simulink model "gm_sampleModel1606_5_sub"  (R2023a)
settings: Solver=VariableStepAuto  StartTime=0.0  StopTime=10.0  RelTol=1e-3
libraries: simulink x3, hdlsllib x3
settings Model: Creator=user1  LastModifiedBy=user1
settings OptimizationCC: BlockReduction=off  ConditionallyExecuteInputs=off
settings DebuggingCC: InheritedTsInSrcMsg=none

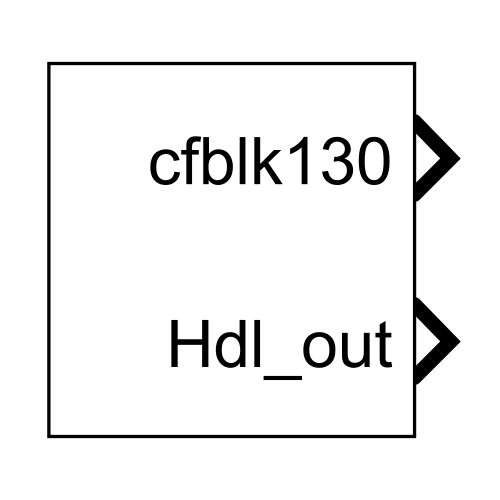
[thumbnail: Simulink's stored preview of the top-level diagram]
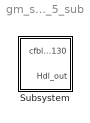
== system gm_sampleModel1606_5_sub ==
  Subsystem : Subsystem

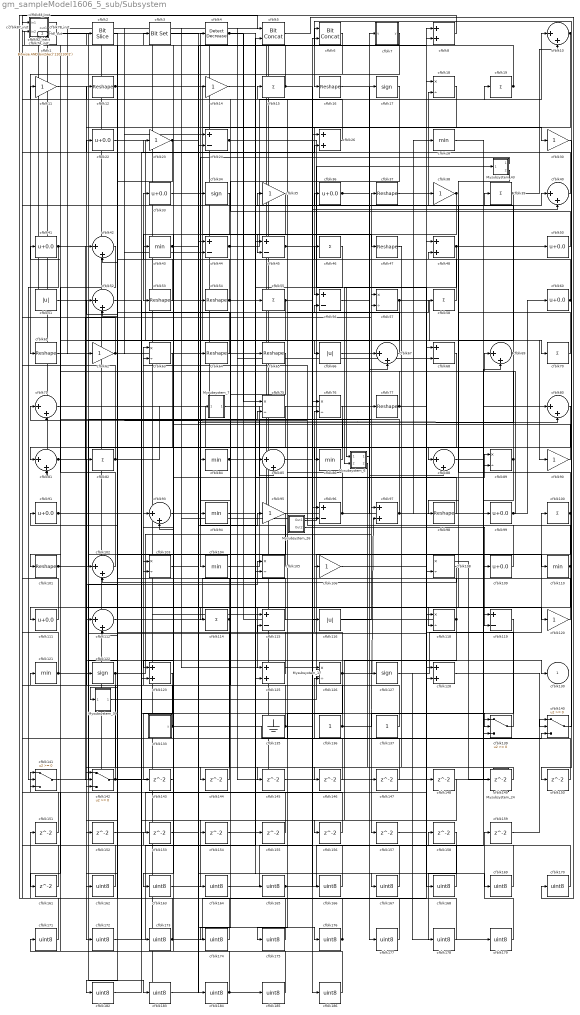
== system gm_sampleModel1606_5_sub/Subsystem ==
  Mysubsystem_17 : Subsystem
  Mysubsystem_24 : Subsystem
  Mysubsystem_26 : Subsystem
  Mysubsystem_39 : Subsystem
  Mysubsystem_43 : Subsystem
  Mysubsystem_6 : Subsystem
  Mysubsystem_7 : Subsystem
  cfblk1 : simulink/Logic and Bit Operations/Bitwise Operator  logicop=AND  UseBitMask=on  BitMask=bin2dec('11011001')  BitMaskRealWorld=Stored Integer
      settings: LibrarySourceBlock=|
      | hdlsllib/Logic and Bit
      | Operations/Bitwise
      | Operator
  cfblk{10,40,42,52,67,69,71,80..81,85,88,93,102,112} (14 alike) : Sum  Inputs=|++  OutDataTypeStr=uint8
  cfblk{15,19,39,46,55,58,70,82,100,114} (10 alike) : Sum  Inputs=+  OutDataTypeStr=uint8
  cfblk{12,16,37,47,53..54,61,64..65,77,98,101} (12 alike) : Reshape
  cfblk{18,57,63,75..76,89,103,105,108,118,126} (11 alike) : Product  Inputs=*/  OutDataTypeStr=uint8  RndMeth=Zero  SaturateOnIntegerOverflow=on
  cfblk{28,43,84,86,94,104,110,121} (8 alike) : MinMax  OutDataTypeStr=uint8
  cfblk{11,14,23,30,35,38,62,90,95,106,120} (11 alike) : Gain  OutDataTypeStr=uint8
  cfblk107_inst : Subsystem
  cfblk{22,33,36,41,50,60,91,99,109,111} (10 alike) : Bias  Bias=0.0  SaturateOnIntegerOverflow=off
  cfblk113_inst : Subsystem
  cfblk{24,44..45,56,68,96,115,119} (8 alike) : Sum  Inputs=+-  OutDataTypeStr=uint8
  cfblk116 : Abs  OutDataTypeStr=uint8  SaturateOnIntegerOverflow=off
  cfblk{17,34,122,127} (4 alike) : Signum
  cfblk{8,26,48,97,123,125,128} (7 alike) : Sum  OutDataTypeStr=uint8
  cfblk133 : Subsystem  mask(Counter Limited){uplimit=double(7), tsamp=double(-1)}
      mask prompts: uplimit "Simulink:masks:UpperLimit_MP"; tsamp "Simulink:masks:SampleTime_MP"
      mask help: Simulink:masks:CounterLimited_MD
      mask init:
      | nbits = double(8);
      | tsamp = double(-1);
      | uplimit = double(7);
  cfblk135 : Ground
  cfblk136 : Constant  OutDataTypeStr=uint8  SampleTime=-1
  cfblk137 : Constant  OutDataTypeStr=uint8  SampleTime=-1
  cfblk{139..142} (4 alike) : Switch  OutDataTypeStr=uint8  SaturateOnIntegerOverflow=off  InputSameDT=off
  cfblk{143..159,161} (18 alike) : Delay  SampleTime=1
  cfblk{162..179,182..186} (23 alike) : DataTypeConversion  OutDataTypeStr=uint8  SaturateOnIntegerOverflow=off  RndMeth=Floor
  cfblk2 : hdlsllib/Logic and Bit Operations/Bit Slice  lidx=7  ridx=0
  cfblk20_inst : Subsystem
  cfblk21_inst : Subsystem
  cfblk25_inst : Subsystem
  cfblk27_inst : Subsystem
  cfblk29_inst : Subsystem
  cfblk3 : simulink/Logic and Bit Operations/Bit Set  iBit=0
      settings: LibrarySourceBlock=|
      | hdlsllib/Logic and Bit
      | Operations/Bit Set
  cfblk32_inst : Subsystem
  cfblk4 : simulink/Logic and Bit Operations/Detect Decrease  vinit=0.0  OutDataTypeStr=uint8
      settings: LibrarySourceBlock=|
      | hdlsllib/Logic and Bit
      | Operations/Detect
      | Decrease
  cfblk5 : hdlsllib/Logic and Bit Operations/Bit Concat  numInputs=2
  cfblk51 : Abs  OutDataTypeStr=uint8  SaturateOnIntegerOverflow=off
  cfblk6 : hdlsllib/Logic and Bit Operations/Bit Concat  numInputs=2
  cfblk66 : Abs  OutDataTypeStr=uint8  SaturateOnIntegerOverflow=off
  cfblk7 : Subsystem  mask(Compare To Constant){relop=<=, const=double(3), OutDataTypeStr=uint8, ZeroCross=on}
      mask prompts: relop "Simulink:masks:Operator_MP"; const "Simulink:masks:ConstantValue_MP"; OutDataTypeStr "Simulink:masks:OutputDataType_MP"; ZeroCross "Simulink:masks:EnableZerocrossingDetection_MP"
      mask help: Simulink:masks:CompareToConstant_MD
      mask init:
      | OutDataTypeStr = 'uint8';
      | ZeroCross = 'on';
      | blkName = 'sampleModel1606_5_sub/Subsystem/cfblk7';
      | const = double(3);
      | const_str = '3.0';
      | const_val = double(3);
      | relop = '<=';
      | setValue = 'fixdt(0, 8)';
      | str = '<= 3';
      mask TypeOptions relop: == | ~= | < | <= | >= | >
      mask TypeOptions OutDataTypeStr: Simulink:masks:uint8 | Simulink:masks:boolean
      mask Callback ZeroCross: sl('zeroCrossEnable', gcbh);
      mask Display: disp(str)
  cfblk74_inst : Subsystem
  cfblk78_inst : Subsystem
  cfblk83_inst : Subsystem
  cfblk87_inst : Subsystem
  cfblk92_inst : Subsystem
  cfblk130 : Outport  OutDataTypeStr=uint8  SampleTime=1  VectorParamsAs1DForOutWhenUnconnected=off
  Hdl_out : Outport  Port=2  OutDataTypeStr=uint8  SampleTime=1
  wires:
  Mysubsystem_17/1(Out1) -> cfblk179/1
  Mysubsystem_24/1(Out1) -> cfblk108/1
  Mysubsystem_26/1(Out1) -> Mysubsystem_43/1(In1)
  Mysubsystem_26/2(Out2) -> cfblk119/2
  Mysubsystem_39/1(Out1) -> Mysubsystem_17/2(In2)
  Mysubsystem_43/1(Out1) -> cfblk104/1
  Mysubsystem_43/2(Out2) -> cfblk118/2
  Mysubsystem_6/1(Out1) -> cfblk145/1
  Mysubsystem_6/2(Out2) -> cfblk146/1
  Mysubsystem_7/1(Out1) -> cfblk85/2
  cfblk1/1 -> cfblk183/1, cfblk108/2
  cfblk10/1 -> cfblk56/1, cfblk172/1
  cfblk100/1 -> cfblk48/2, Mysubsystem_17/1(In1)
  cfblk101/1 -> cfblk75/2, cfblk130/1
  cfblk102/1 -> cfblk107_inst/2(in2)
  cfblk103/1 -> cfblk184/1
  cfblk104/1 -> cfblk37/1
  cfblk105/1 -> cfblk4/1
  cfblk106/1 -> cfblk109/1
  cfblk107_inst/1(out1) -> cfblk81/2, cfblk185/1, cfblk126/1
  cfblk108/1 -> cfblk102/2
  cfblk109/1 -> cfblk63/1
  cfblk11/1 -> cfblk42/1
  cfblk110/1 -> cfblk71/1, cfblk125/1, cfblk111/1
  cfblk111/1 -> cfblk20_inst/2(in2)
  cfblk112/1 -> cfblk26/1
  cfblk113_inst/1(out1) -> cfblk148/1
  cfblk114/1 -> cfblk22/1, cfblk144/1
  cfblk115/1 -> cfblk20_inst/1(in1)
  cfblk116/1 -> cfblk57/1
  cfblk118/1 -> cfblk76/2, cfblk156/1, Hdl_out/1
  cfblk119/1 -> cfblk157/1
  cfblk12/1 -> cfblk66/1, cfblk30/1
  cfblk120/1 -> cfblk76/1
  cfblk121/1 -> cfblk25_inst/2(in2), cfblk105/1
  cfblk122/1 -> cfblk97/1, cfblk142/3
  cfblk123/1 -> cfblk143/1
  cfblk125/1 -> cfblk91/1
  cfblk126/1 -> cfblk175/1, cfblk106/1, cfblk15/1
  cfblk127/1 -> cfblk100/1
  cfblk128/1 -> cfblk140/2
  cfblk133/1(y) -> cfblk140/3, cfblk63/2
  cfblk135/1 -> cfblk186/1, cfblk82/1
  cfblk136/1 -> cfblk97/2, cfblk121/1
  cfblk137/1 -> cfblk54/1
  cfblk139/1 -> cfblk48/1
  cfblk14/1 -> cfblk155/1
  cfblk140/1 -> cfblk16/1
  cfblk141/1 -> cfblk118/1
  cfblk142/1 -> cfblk56/2, cfblk29_inst/2(in2)
  cfblk143/1 -> cfblk1/1
  cfblk144/1 -> cfblk102/1
  cfblk145/1 -> cfblk40/2
  cfblk146/1 -> cfblk126/2
  cfblk147/1 -> cfblk115/2
  cfblk148/1 -> cfblk164/1
  cfblk149/1 -> cfblk142/1
  cfblk15/1 -> cfblk88/1, cfblk21_inst/1(in1)
  cfblk150/1 -> cfblk83_inst/2(in2)
  cfblk151/1 -> cfblk74_inst/2(in2)
  cfblk152/1 -> cfblk68/1
  cfblk153/1 -> cfblk24/2
  cfblk154/1 -> cfblk89/1
  cfblk155/1 -> cfblk78_inst/1(in1)
  cfblk156/1 -> cfblk141/1
  cfblk157/1 -> cfblk128/1
  cfblk158/1 -> cfblk178/1
  cfblk159/1 -> cfblk140/1
  cfblk16/1 -> cfblk177/1
  cfblk161/1 -> cfblk21_inst/2(in2)
  cfblk162/1 -> cfblk74_inst/1(in1)
  cfblk163/1 -> cfblk6/1
  cfblk164/1 -> cfblk6/2
  cfblk165/1 -> cfblk96/1, cfblk69/2
  cfblk166/1 -> cfblk27_inst/1(in1)
  cfblk167/1 -> cfblk27_inst/2(in2)
  cfblk168/1 -> cfblk3/1
  cfblk169/1 -> cfblk158/1
  cfblk17/1 -> cfblk84/1
  cfblk170/1 -> cfblk153/1
  cfblk171/1 -> cfblk5/1
  cfblk172/1 -> cfblk5/2
  cfblk173/1 -> cfblk18/1, cfblk151/1
  cfblk174/1 -> cfblk52/1
  cfblk175/1 -> cfblk52/2
  cfblk176/1 -> cfblk87_inst/1(in1), cfblk78_inst/2(in2)
  cfblk177/1 -> cfblk93/1
  cfblk178/1 -> cfblk93/2
  cfblk179/1 -> cfblk159/1
  cfblk18/1 -> cfblk112/1
  cfblk182/1 -> cfblk123/2
  cfblk183/1 -> cfblk95/1
  cfblk184/1 -> cfblk171/1, cfblk141/3
  cfblk185/1 -> cfblk103/1
  cfblk186/1 -> cfblk103/2
  cfblk19/1 -> cfblk87_inst/2(in2), cfblk113_inst/2(in2)
  cfblk2/1 -> cfblk122/1
  cfblk20_inst/1(out1) -> cfblk64/1
  cfblk21_inst/1(out1) -> cfblk24/1
  cfblk22/1 -> cfblk85/1
  cfblk23/1 -> cfblk112/2, cfblk86/1
  cfblk24/1 -> cfblk128/2, cfblk116/1
  cfblk25_inst/1(out1) -> cfblk99/1, cfblk115/1, cfblk55/1
  cfblk26/1 -> cfblk29_inst/1(in1)
  cfblk27_inst/1(out1) -> cfblk165/1
  cfblk28/1 -> cfblk119/1
  cfblk29_inst/1(out1) -> cfblk113_inst/1(in1)
  cfblk3/1 -> cfblk169/1
  cfblk30/1 -> cfblk150/1
  cfblk32_inst/1(out1) -> cfblk44/2
  cfblk33/1 -> cfblk67/1
  cfblk34/1 -> cfblk53/1
  cfblk35/1 -> cfblk174/1
  cfblk36/1 -> cfblk88/2, cfblk19/1
  cfblk37/1 -> cfblk18/2
  cfblk38/1 -> cfblk45/2, cfblk123/1
  cfblk39/1 -> cfblk98/1, cfblk10/2
  cfblk4/1 -> cfblk167/1, cfblk75/1
  cfblk40/1 -> cfblk25_inst/1(in1)
  cfblk41/1 -> cfblk142/2, cfblk141/2
  cfblk42/1 -> cfblk101/1
  cfblk43/1 -> cfblk80/2, cfblk127/1
  cfblk44/1 -> cfblk10/1, cfblk89/2
  cfblk45/1 -> cfblk47/1, Mysubsystem_6/1(In1)
  cfblk46/1 -> cfblk125/2
  cfblk47/1 -> cfblk147/1
  cfblk48/1 -> cfblk50/1, Mysubsystem_6/2(In2)
  cfblk5/1 -> cfblk170/1
  cfblk50/1 -> cfblk14/1
  cfblk51/1 -> cfblk70/1
  cfblk52/1 -> cfblk173/1
  cfblk53/1 -> cfblk12/1
  cfblk54/1 -> cfblk36/1, cfblk107_inst/1(in1)
  cfblk55/1 -> cfblk166/1, cfblk139/2, Mysubsystem_39/1(In1), cfblk110/1
  cfblk56/1 -> cfblk7/1(u)
  cfblk57/1 -> cfblk90/1, cfblk161/1
  cfblk58/1 -> cfblk46/1
  cfblk6/1 -> cfblk162/1
  cfblk60/1 -> cfblk33/1, cfblk2/1
  cfblk61/1 -> cfblk149/1
  cfblk62/1 -> cfblk32_inst/2(in2), cfblk26/2
  cfblk63/1 -> cfblk81/1
  cfblk64/1 -> cfblk92_inst/1(in1)
  cfblk65/1 -> cfblk114/1
  cfblk66/1 -> cfblk67/2
  cfblk67/1 -> cfblk35/1
  cfblk68/1 -> cfblk163/1
  cfblk69/1 -> cfblk71/2, cfblk32_inst/1(in1)
  cfblk7/1(y) -> cfblk61/1
  cfblk70/1 -> cfblk38/1
  cfblk71/1 -> cfblk168/1
  cfblk74_inst/1(out1) -> cfblk77/1, cfblk51/1
  cfblk75/1 -> cfblk152/1
  cfblk76/1 -> cfblk94/1
  cfblk77/1 -> cfblk8/2, cfblk44/1
  cfblk78_inst/1(out1) -> cfblk65/1
  cfblk8/1 -> cfblk83_inst/1(in1)
  cfblk80/1 -> cfblk105/2
  cfblk81/1 -> cfblk57/2, cfblk120/1
  cfblk82/1 -> cfblk92_inst/2(in2), Mysubsystem_7/1(In1)
  cfblk83_inst/1(out1) -> cfblk96/2
  cfblk84/1 -> cfblk39/1, cfblk58/1
  cfblk85/1 -> cfblk40/1
  cfblk86/1 -> cfblk11/1
  cfblk87_inst/1(out1) -> cfblk62/1, Mysubsystem_24/1(In1)
  cfblk88/1 -> cfblk80/1
  cfblk89/1 -> cfblk41/1, cfblk139/3
  cfblk90/1 -> cfblk43/1
  cfblk91/1 -> cfblk139/1, cfblk154/1
  cfblk92_inst/1(out1) -> cfblk68/2
  cfblk93/1 -> cfblk176/1
  cfblk94/1 -> cfblk8/1
  cfblk95/1 -> cfblk182/1
  cfblk96/1 -> cfblk45/1, cfblk34/1, cfblk17/1
  cfblk97/1 -> cfblk42/2, cfblk28/1
  cfblk98/1 -> cfblk23/1
  cfblk99/1 -> cfblk69/1, cfblk60/1

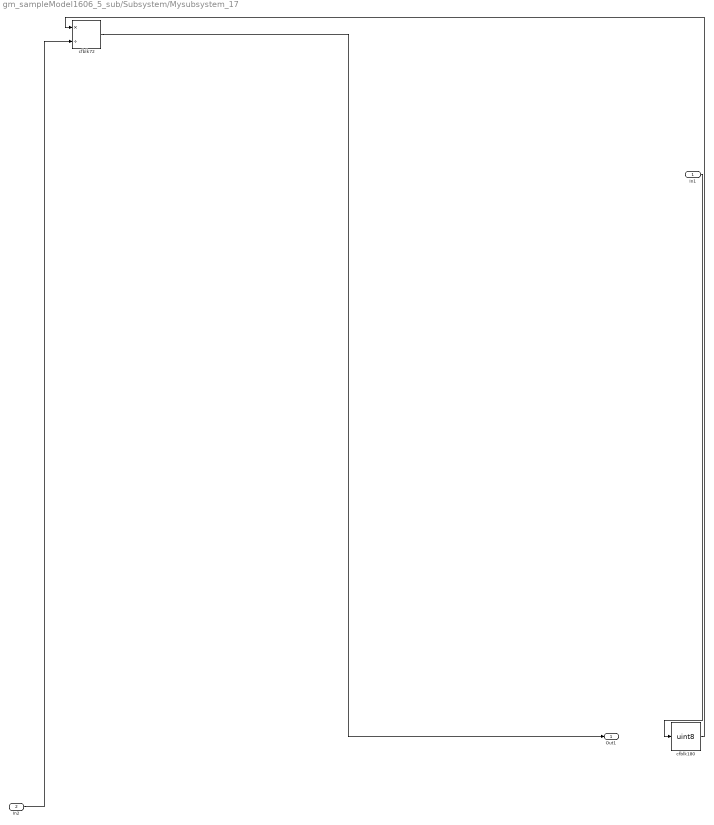
== system gm_sampleModel1606_5_sub/Subsystem/Mysubsystem_17 ==
  In1 : Inport  OutDataTypeStr=uint8  PortDimensions=1  SampleTime=1
  In2 : Inport  Port=2  OutDataTypeStr=uint8  PortDimensions=1  SampleTime=1
  cfblk180 : DataTypeConversion  OutDataTypeStr=uint8  SaturateOnIntegerOverflow=off  RndMeth=Floor
  cfblk72 : Product  Inputs=*/  RndMeth=Zero  SaturateOnIntegerOverflow=on
  Out1 : Outport  SampleTime=1
  wires:
  In1/1 -> cfblk180/1
  In2/1 -> cfblk72/2
  cfblk180/1 -> cfblk72/1
  cfblk72/1 -> Out1/1

== system gm_sampleModel1606_5_sub/Subsystem/Mysubsystem_24 ==
  In1 : Inport  OutDataTypeStr=uint8  PortDimensions=1  SampleTime=1
  cfblk138 : Subsystem
  cfblk160 : Delay  SampleTime=1
  Out1 : Outport  SampleTime=1
  wires:
  In1/1 -> cfblk138/1(In1)
  cfblk138/1(Out1) -> cfblk160/1
  cfblk160/1 -> Out1/1

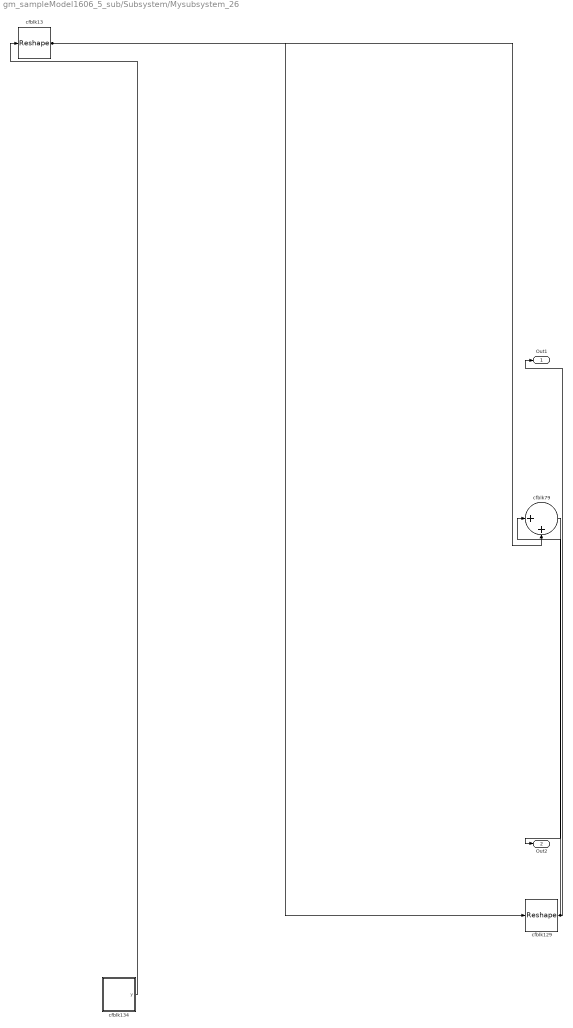
== system gm_sampleModel1606_5_sub/Subsystem/Mysubsystem_26 ==
  cfblk129 : Reshape
  cfblk13 : Reshape
  cfblk134 : Subsystem  mask(Counter Free-Running){NumBits=double(16), tsamp=double(-1)}
      mask prompts: NumBits "Simulink:masks:NumberOfBits_MP"; tsamp "Simulink:masks:SampleTime_MP"
      mask help: Simulink:masks:CounterFreeRunning_MD
  cfblk79 : Sum  Inputs=|++
  Out1 : Outport  SampleTime=1
  Out2 : Outport  Port=2  SampleTime=1
  wires:
  cfblk129/1 -> cfblk79/1, Out1/1
  cfblk13/1 -> cfblk79/2, cfblk129/1
  cfblk134/1(y) -> cfblk13/1
  cfblk79/1 -> Out2/1

== system gm_sampleModel1606_5_sub/Subsystem/Mysubsystem_39 ==
  In1 : Inport  OutDataTypeStr=uint8  PortDimensions=1  SampleTime=1
  cfblk181 : DataTypeConversion  OutDataTypeStr=uint8  SaturateOnIntegerOverflow=off  RndMeth=Floor
  cfblk73 : MinMax
  Out1 : Outport  SampleTime=1
  wires:
  In1/1 -> cfblk73/1
  cfblk181/1 -> Out1/1
  cfblk73/1 -> cfblk181/1

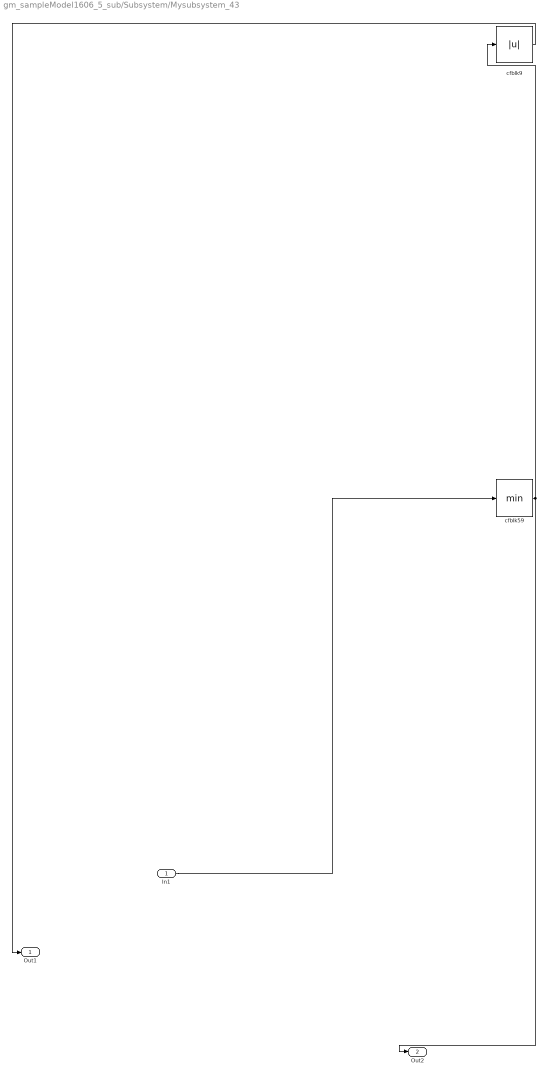
== system gm_sampleModel1606_5_sub/Subsystem/Mysubsystem_43 ==
  In1 : Inport  OutDataTypeStr=uint16  PortDimensions=1  SampleTime=1
  cfblk59 : MinMax
  cfblk9 : Abs  SaturateOnIntegerOverflow=off
  Out1 : Outport  SampleTime=1
  Out2 : Outport  Port=2  SampleTime=1
  wires:
  In1/1 -> cfblk59/1
  cfblk59/1 -> cfblk9/1, Out2/1
  cfblk9/1 -> Out1/1

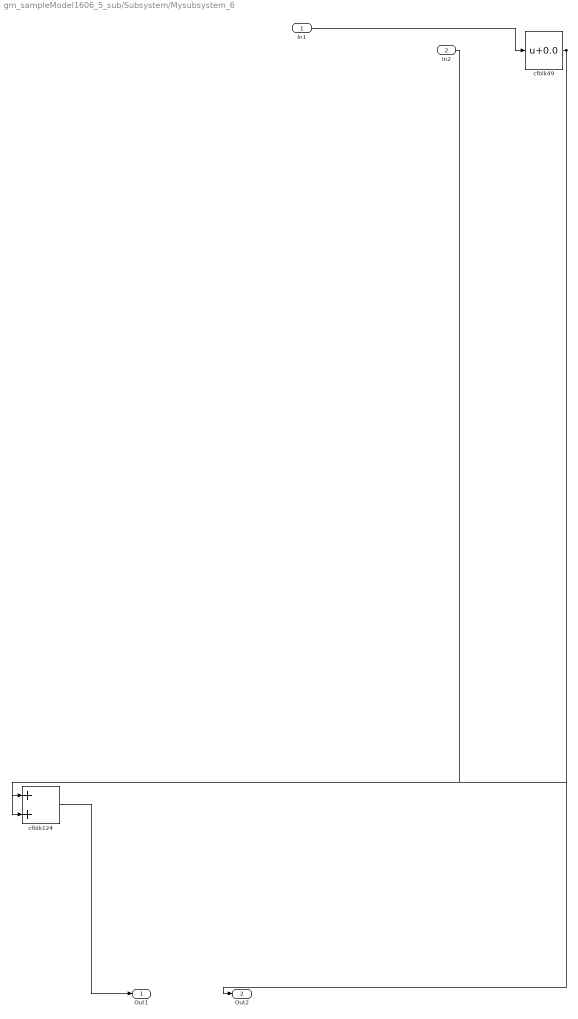
== system gm_sampleModel1606_5_sub/Subsystem/Mysubsystem_6 ==
  In1 : Inport  OutDataTypeStr=uint8  PortDimensions=1  SampleTime=1
  In2 : Inport  Port=2  OutDataTypeStr=uint8  PortDimensions=1  SampleTime=1
  cfblk124 : Sum
  cfblk49 : Bias  Bias=0.0  SaturateOnIntegerOverflow=off
  Out1 : Outport  SampleTime=1
  Out2 : Outport  Port=2  SampleTime=1
  wires:
  In1/1 -> cfblk49/1
  In2/1 -> cfblk124/2
  cfblk124/1 -> Out1/1
  cfblk49/1 -> cfblk124/1, Out2/1

== system gm_sampleModel1606_5_sub/Subsystem/Mysubsystem_7 ==
  In1 : Inport  OutDataTypeStr=uint8  PortDimensions=1  SampleTime=1
  cfblk117 : MinMax
  cfblk31 : Sum  Inputs=+
  Out1 : Outport  SampleTime=1
  wires:
  In1/1 -> cfblk117/1
  cfblk117/1 -> cfblk31/1
  cfblk31/1 -> Out1/1

== system gm_sampleModel1606_5_sub/Subsystem/cfblk107_inst ==
  in1 : Inport  OutDataTypeStr=uint8  SampleTime=1
  in2 : Inport  Port=2  OutDataTypeStr=uint8  SampleTime=1
  mul_cfblk107_dotp_mulcomp : Product  Inputs=**  OutDataTypeStr=uint8  SampleTime=1
  out1 : Outport  OutDataTypeStr=uint8  SampleTime=1
  wires:
  in1/1 -> mul_cfblk107_dotp_mulcomp/1
  in2/1 -> mul_cfblk107_dotp_mulcomp/2
  mul_cfblk107_dotp_mulcomp/1 -> out1/1

== system gm_sampleModel1606_5_sub/Subsystem/cfblk113_inst ==
  in1 : Inport  OutDataTypeStr=uint8  SampleTime=1
  in2 : Inport  Port=2  OutDataTypeStr=uint8  SampleTime=1
  mul_cfblk113_dotp_mulcomp : Product  Inputs=**  OutDataTypeStr=uint8  SampleTime=1
  out1 : Outport  OutDataTypeStr=uint8  SampleTime=1
  wires:
  in1/1 -> mul_cfblk113_dotp_mulcomp/1
  in2/1 -> mul_cfblk113_dotp_mulcomp/2
  mul_cfblk113_dotp_mulcomp/1 -> out1/1

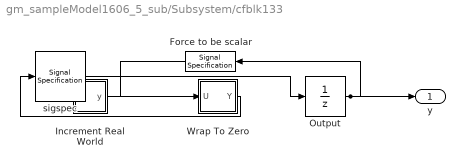
== system gm_sampleModel1606_5_sub/Subsystem/cfblk133 ==
  Force to be scalar : SignalSpecification  DisableCoverage=on  Dimensions=1
  Increment Real World : Subsystem  mask(Real World Value Increment){}
      mask help: Simulink:masks:RealWorldValueIncrement_MD
      mask Display: disp('V++')
  Output : UnitDelay  InitialCondition=0.0  SampleTime=tsamp  HasFrameUpgradeWarning=on
  Wrap To Zero : Subsystem  mask(Wrap To Zero){Threshold=double(7)}
      mask prompts: Threshold "Simulink:masks:Threshold_MP"
      mask help: Simulink:masks:WrapToZero_MD
  sigspec : SignalSpecification  OutDataTypeStr=uint8  Dimensions=1
  y : Outport  SampleTime=1
  wires:
  Force to be scalar/1 -> Increment Real World/1(u)
  Increment Real World/1(y) -> Wrap To Zero/1(U)
  Output/1 -> Force to be scalar/1, y/1
  Wrap To Zero/1(Y) -> sigspec/1
  sigspec/1 -> Output/1

== system gm_sampleModel1606_5_sub/Subsystem/cfblk20_inst ==
  in1 : Inport  OutDataTypeStr=uint8  SampleTime=1
  in2 : Inport  Port=2  OutDataTypeStr=uint8  SampleTime=1
  mul_cfblk20_dotp_mulcomp : Product  Inputs=**  OutDataTypeStr=uint8  SampleTime=1
  out1 : Outport  OutDataTypeStr=uint8  SampleTime=1
  wires:
  in1/1 -> mul_cfblk20_dotp_mulcomp/1
  in2/1 -> mul_cfblk20_dotp_mulcomp/2
  mul_cfblk20_dotp_mulcomp/1 -> out1/1

== system gm_sampleModel1606_5_sub/Subsystem/cfblk21_inst ==
  in1 : Inport  OutDataTypeStr=uint8  SampleTime=1
  in2 : Inport  Port=2  OutDataTypeStr=uint8  SampleTime=1
  mul_cfblk21_dotp_mulcomp : Product  Inputs=**  OutDataTypeStr=uint8  SampleTime=1
  out1 : Outport  OutDataTypeStr=uint8  SampleTime=1
  wires:
  in1/1 -> mul_cfblk21_dotp_mulcomp/1
  in2/1 -> mul_cfblk21_dotp_mulcomp/2
  mul_cfblk21_dotp_mulcomp/1 -> out1/1

== system gm_sampleModel1606_5_sub/Subsystem/cfblk25_inst ==
  in1 : Inport  OutDataTypeStr=uint8  SampleTime=1
  in2 : Inport  Port=2  OutDataTypeStr=uint8  SampleTime=1
  mul_cfblk25_dotp_mulcomp : Product  Inputs=**  OutDataTypeStr=uint8  SampleTime=1
  out1 : Outport  OutDataTypeStr=uint8  SampleTime=1
  wires:
  in1/1 -> mul_cfblk25_dotp_mulcomp/1
  in2/1 -> mul_cfblk25_dotp_mulcomp/2
  mul_cfblk25_dotp_mulcomp/1 -> out1/1

== system gm_sampleModel1606_5_sub/Subsystem/cfblk27_inst ==
  in1 : Inport  OutDataTypeStr=uint8  SampleTime=1
  in2 : Inport  Port=2  OutDataTypeStr=uint8  SampleTime=1
  mul_cfblk27_dotp_mulcomp : Product  Inputs=**  OutDataTypeStr=uint8  SampleTime=1
  out1 : Outport  OutDataTypeStr=uint8  SampleTime=1
  wires:
  in1/1 -> mul_cfblk27_dotp_mulcomp/1
  in2/1 -> mul_cfblk27_dotp_mulcomp/2
  mul_cfblk27_dotp_mulcomp/1 -> out1/1

== system gm_sampleModel1606_5_sub/Subsystem/cfblk29_inst ==
  in1 : Inport  OutDataTypeStr=uint8  SampleTime=1
  in2 : Inport  Port=2  OutDataTypeStr=uint8  SampleTime=1
  mul_cfblk29_dotp_mulcomp : Product  Inputs=**  OutDataTypeStr=uint8  SampleTime=1
  out1 : Outport  OutDataTypeStr=uint8  SampleTime=1
  wires:
  in1/1 -> mul_cfblk29_dotp_mulcomp/1
  in2/1 -> mul_cfblk29_dotp_mulcomp/2
  mul_cfblk29_dotp_mulcomp/1 -> out1/1

== system gm_sampleModel1606_5_sub/Subsystem/cfblk32_inst ==
  in1 : Inport  OutDataTypeStr=uint8  SampleTime=1
  in2 : Inport  Port=2  OutDataTypeStr=uint8  SampleTime=1
  mul_cfblk32_dotp_mulcomp : Product  Inputs=**  OutDataTypeStr=uint8  SampleTime=1
  out1 : Outport  OutDataTypeStr=uint8  SampleTime=1
  wires:
  in1/1 -> mul_cfblk32_dotp_mulcomp/1
  in2/1 -> mul_cfblk32_dotp_mulcomp/2
  mul_cfblk32_dotp_mulcomp/1 -> out1/1

== system gm_sampleModel1606_5_sub/Subsystem/cfblk7 ==
  u : Inport  OutDataTypeStr=uint8  SampleTime=1
  Compare : RelationalOperator  Operator=<=  OutDataTypeStr=fixdt(0, 8)
  Constant : Constant  DisableCoverage=on  Value=const  OutDataTypeStr=Inherit: Inherit via back propagation  SampleTime=-1
  y : Outport  SampleTime=1
  wires:
  u/1 -> Compare/1
  Compare/1 -> y/1
  Constant/1 -> Compare/2

== system gm_sampleModel1606_5_sub/Subsystem/cfblk74_inst ==
  in1 : Inport  OutDataTypeStr=uint8  SampleTime=1
  in2 : Inport  Port=2  OutDataTypeStr=uint8  SampleTime=1
  mul_cfblk74_dotp_mulcomp : Product  Inputs=**  OutDataTypeStr=uint8  SampleTime=1
  out1 : Outport  OutDataTypeStr=uint8  SampleTime=1
  wires:
  in1/1 -> mul_cfblk74_dotp_mulcomp/1
  in2/1 -> mul_cfblk74_dotp_mulcomp/2
  mul_cfblk74_dotp_mulcomp/1 -> out1/1

== system gm_sampleModel1606_5_sub/Subsystem/cfblk78_inst ==
  in1 : Inport  OutDataTypeStr=uint8  SampleTime=1
  in2 : Inport  Port=2  OutDataTypeStr=uint8  SampleTime=1
  mul_cfblk78_dotp_mulcomp : Product  Inputs=**  OutDataTypeStr=uint8  SampleTime=1
  out1 : Outport  OutDataTypeStr=uint8  SampleTime=1
  wires:
  in1/1 -> mul_cfblk78_dotp_mulcomp/1
  in2/1 -> mul_cfblk78_dotp_mulcomp/2
  mul_cfblk78_dotp_mulcomp/1 -> out1/1

== system gm_sampleModel1606_5_sub/Subsystem/cfblk83_inst ==
  in1 : Inport  OutDataTypeStr=uint8  SampleTime=1
  in2 : Inport  Port=2  OutDataTypeStr=uint8  SampleTime=1
  mul_cfblk83_dotp_mulcomp : Product  Inputs=**  OutDataTypeStr=uint8  SampleTime=1
  out1 : Outport  OutDataTypeStr=uint8  SampleTime=1
  wires:
  in1/1 -> mul_cfblk83_dotp_mulcomp/1
  in2/1 -> mul_cfblk83_dotp_mulcomp/2
  mul_cfblk83_dotp_mulcomp/1 -> out1/1

== system gm_sampleModel1606_5_sub/Subsystem/cfblk87_inst ==
  in1 : Inport  OutDataTypeStr=uint8  SampleTime=1
  in2 : Inport  Port=2  OutDataTypeStr=uint8  SampleTime=1
  mul_cfblk87_dotp_mulcomp : Product  Inputs=**  OutDataTypeStr=uint8  SampleTime=1
  out1 : Outport  OutDataTypeStr=uint8  SampleTime=1
  wires:
  in1/1 -> mul_cfblk87_dotp_mulcomp/1
  in2/1 -> mul_cfblk87_dotp_mulcomp/2
  mul_cfblk87_dotp_mulcomp/1 -> out1/1

== system gm_sampleModel1606_5_sub/Subsystem/cfblk92_inst ==
  in1 : Inport  OutDataTypeStr=uint8  SampleTime=1
  in2 : Inport  Port=2  OutDataTypeStr=uint8  SampleTime=1
  mul_cfblk92_dotp_mulcomp : Product  Inputs=**  OutDataTypeStr=uint8  SampleTime=1
  out1 : Outport  OutDataTypeStr=uint8  SampleTime=1
  wires:
  in1/1 -> mul_cfblk92_dotp_mulcomp/1
  in2/1 -> mul_cfblk92_dotp_mulcomp/2
  mul_cfblk92_dotp_mulcomp/1 -> out1/1

== system gm_sampleModel1606_5_sub/Subsystem/Mysubsystem_24/cfblk138 ==
  In1 : Inport  OutDataTypeStr=uint8  PortDimensions=1  SampleTime=1
  Out1 : Outport  SampleTime=1
  wires:
  In1/1 -> Out1/1

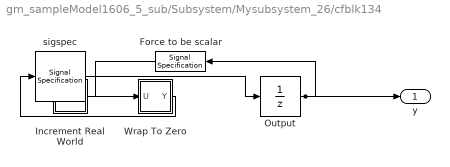
== system gm_sampleModel1606_5_sub/Subsystem/Mysubsystem_26/cfblk134 ==
  Force to be scalar : SignalSpecification  DisableCoverage=on  Dimensions=1
  Increment Real World : Subsystem  mask(Real World Value Increment){}
      mask help: Simulink:masks:RealWorldValueIncrement_MD
      mask Display: disp('V++')
  Output : UnitDelay  InitialCondition=0.0  SampleTime=tsamp  HasFrameUpgradeWarning=on
  Wrap To Zero : Subsystem  mask(Wrap To Zero){Threshold=double(65535)}
      mask prompts: Threshold "Simulink:masks:Threshold_MP"
      mask help: Simulink:masks:WrapToZero_MD
  sigspec : SignalSpecification  OutDataTypeStr=uint16  Dimensions=1
  y : Outport  SampleTime=1
  wires:
  Force to be scalar/1 -> Increment Real World/1(u)
  Increment Real World/1(y) -> Wrap To Zero/1(U)
  Output/1 -> Force to be scalar/1, y/1
  Wrap To Zero/1(Y) -> sigspec/1
  sigspec/1 -> Output/1

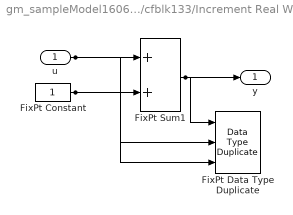
== system gm_sampleModel1606_5_sub/Subsystem/cfblk133/Increment Real World ==
  u : Inport  OutDataTypeStr=uint8  SampleTime=1
  FixPt Constant : Constant  DisableCoverage=on  OutDataTypeStr=Inherit: Inherit via back propagation  SampleTime=-1
  FixPt Data Type Duplicate : DataTypeDuplicate  DisableCoverage=on  NumInputPorts=3
  FixPt Sum1 : Sum  InputSameDT=on  OutDataTypeStr=Inherit: Inherit via back propagation  LockScale=on
  y : Outport  SampleTime=1
  wires:
  u/1 -> FixPt Sum1/1, FixPt Data Type Duplicate/2
  FixPt Constant/1 -> FixPt Sum1/2, FixPt Data Type Duplicate/3
  FixPt Sum1/1 -> FixPt Data Type Duplicate/1, y/1

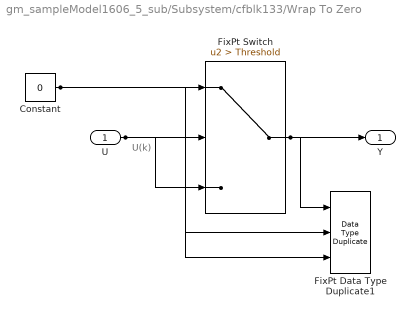
== system gm_sampleModel1606_5_sub/Subsystem/cfblk133/Wrap To Zero ==
  note: U(k)
  U : Inport  OutDataTypeStr=uint8  SampleTime=1
  Constant : Constant  DisableCoverage=on  Value=0  OutDataTypeStr=Inherit: Inherit via back propagation  SampleTime=-1
  FixPt Data Type Duplicate1 : DataTypeDuplicate  DisableCoverage=on  NumInputPorts=3
  FixPt Switch : Switch  Criteria=u2 > Threshold  Threshold=Threshold  OutDataTypeStr=Inherit: Inherit via back propagation  ZeroCross=off  SaturateOnIntegerOverflow=off  InputSameDT=off
  Y : Outport  SampleTime=1
  wires:
  U/1 -> FixPt Switch/3, FixPt Switch/2, FixPt Data Type Duplicate1/2
  Constant/1 -> FixPt Switch/1, FixPt Data Type Duplicate1/3
  FixPt Switch/1 -> FixPt Data Type Duplicate1/1, Y/1

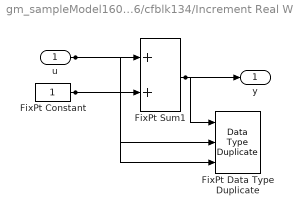
== system gm_sampleModel1606_5_sub/Subsystem/Mysubsystem_26/cfblk134/Increment Real World ==
  u : Inport  OutDataTypeStr=uint16  SampleTime=1
  FixPt Constant : Constant  DisableCoverage=on  OutDataTypeStr=Inherit: Inherit via back propagation  SampleTime=-1
  FixPt Data Type Duplicate : DataTypeDuplicate  DisableCoverage=on  NumInputPorts=3
  FixPt Sum1 : Sum  InputSameDT=on  OutDataTypeStr=Inherit: Inherit via back propagation  LockScale=on
  y : Outport  SampleTime=1
  wires:
  u/1 -> FixPt Sum1/1, FixPt Data Type Duplicate/2
  FixPt Constant/1 -> FixPt Sum1/2, FixPt Data Type Duplicate/3
  FixPt Sum1/1 -> FixPt Data Type Duplicate/1, y/1

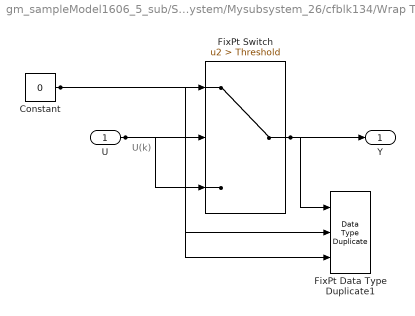
== system gm_sampleModel1606_5_sub/Subsystem/Mysubsystem_26/cfblk134/Wrap To Zero ==
  note: U(k)
  U : Inport  OutDataTypeStr=uint16  SampleTime=1
  Constant : Constant  DisableCoverage=on  Value=0  OutDataTypeStr=Inherit: Inherit via back propagation  SampleTime=-1
  FixPt Data Type Duplicate1 : DataTypeDuplicate  DisableCoverage=on  NumInputPorts=3
  FixPt Switch : Switch  Criteria=u2 > Threshold  Threshold=Threshold  OutDataTypeStr=Inherit: Inherit via back propagation  ZeroCross=off  SaturateOnIntegerOverflow=off  InputSameDT=off
  Y : Outport  SampleTime=1
  wires:
  U/1 -> FixPt Switch/3, FixPt Switch/2, FixPt Data Type Duplicate1/2
  Constant/1 -> FixPt Switch/1, FixPt Data Type Duplicate1/3
  FixPt Switch/1 -> FixPt Data Type Duplicate1/1, Y/1
